simulink model "motion_with_control"  (R2020b)
settings: Solver=FixedStepDiscrete  StartTime=0.0  StopTime=inf  FixedStep=0.001  RelTol=1e-3  EnableMultiTasking=on
PreLoadFcn:
  | demos_common_configs();
undefined symbols (not defined in the file): DiscIntNeverNeededParam
libraries: franka_simulink_library_misc x5, franka_simulink_library x4
settings Model: SimulationMode=external  ExtModeTrigDuration=10000  Creator=vasi_ko  LastModifiedBy=kvasios
settings DataIOCC: LimitDataPoints=on  SaveFormat=Array  ReturnWorkspaceOutputs=off
settings OptimizationCC: DefaultParameterBehavior=Inlined  EnhancedBackFolding=on  PassReuseOutputArgsAs=Individual arguments  ZeroExternalMemoryAtStartup=off  ZeroInternalMemoryAtStartup=off  OptimizeBlockOrder=speed  DifferentSizesBufferReuse=on  OptimizationCustomize=off  EfficientTunableParamExpr=on
settings DebuggingCC: SolverPrmCheckMsg=warning  ParameterTunabilityLossMsg=error  SFUnexpectedBacktrackingDiag=warning  SFNoUnconditionalDefaultTransitionDiag=warning  SFExecutionAtInitializationDiag=none  ArithmeticOperatorsInVariantConditions=warning
settings HardwareCC: ProdBitPerLong=64  ProdHWDeviceType=Intel->x86-64 (Linux 64)
settings ModelReferenceCC: PropagateSignalLabelsOutOfModel=off
settings SFSimCC: SimUseLocalCustomCode=off  MATLABDynamicMemAlloc=off  CustomCodeUndefinedFunction=UseInterfaceOnly  SimTargetLang=C++
settings RTWCC: Description=Embedded Coder  SystemTargetFile=franka_emika_panda.tlc  GenCodeOnly=on  TemplateMakefile=ert_default_tmf  RTWVerbose=off  RTWUseLocalCustomCode=off  Toolchain=Franka Simulink | gmake (64-bit linux)  BuildConfiguration=Faster Runs  IncludeHyperlinkInReport=on  TargetLang=C++
settings CodeAppCC: ForceParamTrailComments=on  IgnoreCustomStorageClasses=off  OperatorAnnotations=on  SimulinkDataObjDesc=on  SFDataObjDesc=on  InsertBlockDesc=on
settings STFCustomTargetCC: TargetLangStandard=C99 (ISO)  MultiwordLength=256  GenerateSampleERTMain=on  ModelReferenceCompliant=off  ConcurrentExecutionCompliant=off  CombineOutputUpdateFcns=on  ERTCustomFileBanners=on  SupportNonInlinedSFcns=off  RemoveResetFunc=on  MATLABClassNameForMDSCustomization=Simulink.SoftwareTarget.ERTCustomization  GRTInterface=off  UseToolchainInfoCompliant=on  SystemTargetFile=franka_emika_panda.tlc
settings ERTTargetCC: TargetLangStandard=C99 (ISO)  GenerateSampleERTMain=on  ModelReferenceCompliant=off  ParMdlRefBuildCompliant=off  CompOptLevelCompliant=off  ConcurrentExecutionCompliant=off  SupportContinuousTime=on  ModelStepFunctionPrototypeControlCompliant=off  InlinedParameterPlacement=NonHierarchical  ERTCustomFileTemplate=franka_emika_panda_file_process.tlc
settings ConfigComp: CovMetricSettings=dw  CovSaveCumulativeToWorkspaceVar=on  CovSaveSingleToWorkspaceVar=on  CovExternalEMLEnable=off  CovSFcnEnable=off

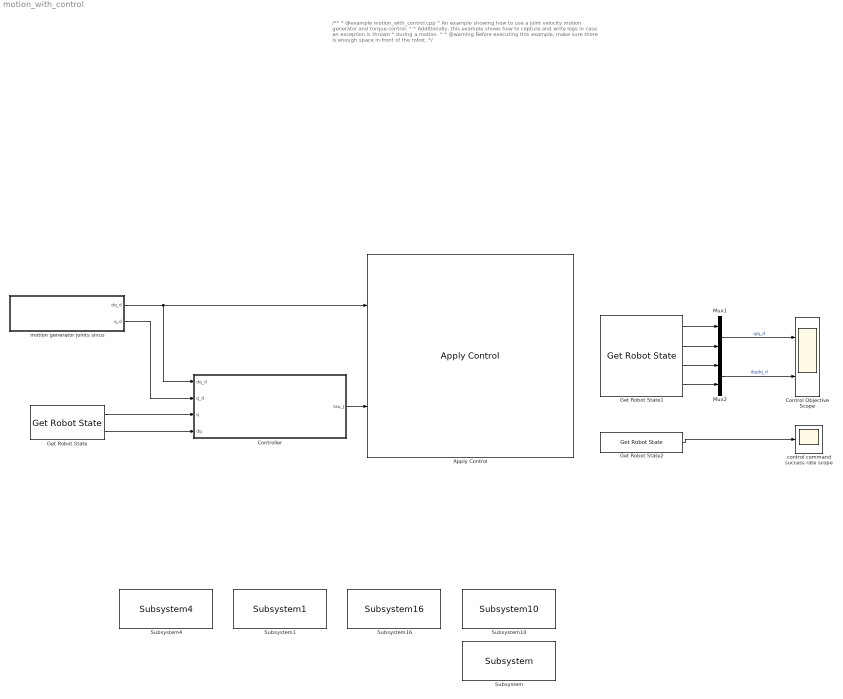
== system motion_with_control ==
  note: /**
      |  * @example motion_with_control.cpp
      |  * An example showing how to use a joint velocity motion generator and torque control.
      |  *
      |  * Additionally, this example shows how to capture and write logs in case an exception is thrown
      |  * during a motion.
      |  *
      |  * @warning Before executing this example, make sure there is enough space in front of the robot.
      |  */
  Apply Control : franka_simulink_library/Apply Control  robot_ip=robot_ip  gripper_attached=off  control_mode=Torque Control - Joint Velocities  controller_choice=Joint Impedance Controller  elbow_control=on  collision_thresholds=collision_behavior  joint_impedance=joint_impedance  cartesian_impedance=cartesian_impedance  load_inertia=load_inertia  EE_T_K=EE_T_K  init_joint_configuration_req=on  init_joint_configuration=q_init
      settings: SourceProductName=Franka Emika
  Control Objective Scope : Scope  NumInputPorts=2
  Controller : Subsystem
      mask Display:
      | % pos = get_param(gcb, 'Position');
      | 
      | disp('{\bf\fontsize{18}PD Controller}', 'texmode','on');
      | 
      | block_icon('Controller')
      | 
      | port_label('output',1,'tau_J_d');
      | 
      | port_label('input',2,'q_d');
      | port_label('input',1,'dq_d');
      | port_label('input',3,'q');
      | port_label('input',4,'dq');
  Get Robot State : franka_simulink_library/Get Robot State  robot_ip=robot_ip  signals_requested='q dq'
      settings: SourceProductName=Franka Emika
  Get Robot State1 : franka_simulink_library/Get Robot State  robot_ip=robot_ip  signals_requested='q q_d dq dq_d'
      settings: SourceProductName=Franka Emika
  Get Robot State2 : franka_simulink_library/Get Robot State  robot_ip=robot_ip  signals_requested='control_command_success_rate'
      settings: SourceProductName=Franka Emika
  Mux1 : Mux  Inputs=2
  Mux2 : Mux  Inputs=2
  Subsystem : franka_simulink_library_misc/Subsystem  SystemSampleTime=-1  VariantActivationTime=update diagram  Latency=0  AutoFrameSizeCalculation=off
  Subsystem1 : franka_simulink_library_misc/Subsystem1  SystemSampleTime=-1  VariantActivationTime=update diagram  Latency=0  AutoFrameSizeCalculation=off
  Subsystem10 : franka_simulink_library_misc/Subsystem10  SystemSampleTime=-1  VariantActivationTime=update diagram  Latency=0  AutoFrameSizeCalculation=off
  Subsystem16 : franka_simulink_library_misc/Subsystem16  SystemSampleTime=-1  VariantActivationTime=update diagram  Latency=0  AutoFrameSizeCalculation=off
  Subsystem4 : franka_simulink_library_misc/Subsystem4  SystemSampleTime=-1  VariantActivationTime=update diagram  Latency=0  AutoFrameSizeCalculation=off
  control command success rate scope : Scope
  motion generator joints sinus : Subsystem
      mask Display:
      | pos = get_param(gcb, 'Position');
      | width = pos(3) - pos(1);
      | x = [0:width];
      | y = sin(x/180*pi);
      | % Parameters 'm' and 'b' must be defined in 'Parameters & Dialog' pane.
      | plot(x,y );
      | 
      | port_label('output',1,'dq_d');
      | port_label('output',2,'q_d');
  wires:
  motion generator joints sinus/1(dq_d) -> Controller/1(dq_d), Apply Control/1
  motion generator joints sinus/2(q_d) -> Controller/2(q_d)
  Controller/1(tau_J) -> Apply Control/2
  Mux2/1 -> Control Objective Scope/2  "dq/dq_d"
  Get Robot State/2 -> Controller/4(dq)
  Mux1/1 -> Control Objective Scope/1  "q/q_d"
  Get Robot State/1 -> Controller/3(q)
  Get Robot State1/1 -> Mux1/1
  Get Robot State1/2 -> Mux1/2
  Get Robot State1/3 -> Mux2/1
  Get Robot State1/4 -> Mux2/2
  Get Robot State2/1 -> control command success rate scope/1

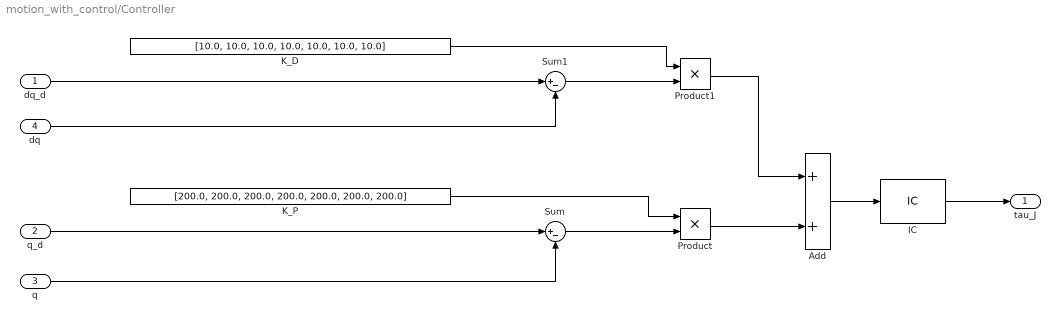
== system motion_with_control/Controller ==
  dq_d : Inport
  q_d : Inport  Port=2
  q : Inport  Port=3
  dq : Inport  Port=4
  Add : Sum
  IC : InitialCondition  Value=zeros(1,7)
  K_D : Constant  Value=[10.0, 10.0, 10.0, 10.0, 10.0, 10.0, 10.0]  VectorParams1D=off  SampleTime=-1
  K_P : Constant  Value=[200.0, 200.0, 200.0, 200.0, 200.0, 200.0, 200.0]  VectorParams1D=off  SampleTime=-1
  Product : Product
  Product1 : Product
  Sum : Sum  Inputs=|+-
  Sum1 : Sum  Inputs=|+-
  tau_J : Outport  VectorParamsAs1DForOutWhenUnconnected=off
  wires:
  IC/1 -> tau_J/1
  Add/1 -> IC/1
  Sum1/1 -> Product1/2
  dq/1 -> Sum1/2
  q_d/1 -> Sum/1
  dq_d/1 -> Sum1/1
  Product1/1 -> Add/1
  Product/1 -> Add/2
  K_D/1 -> Product1/1
  K_P/1 -> Product/1
  Sum/1 -> Product/2
  q/1 -> Sum/2

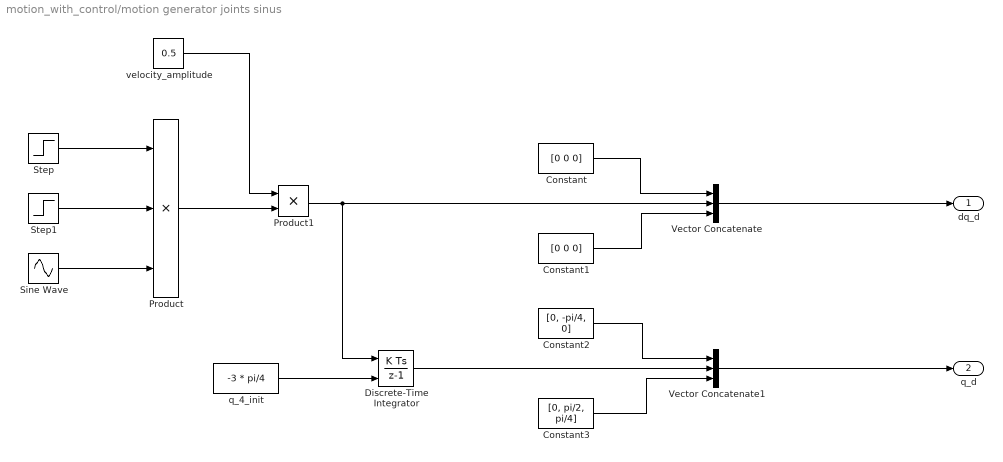
== system motion_with_control/motion generator joints sinus ==
  Constant : Constant  Value=[0 0 0]  VectorParams1D=off
  Constant1 : Constant  Value=[0 0 0]  VectorParams1D=off
  Constant2 : Constant  Value=[0, -pi/4, 0]  VectorParams1D=off
  Constant3 : Constant  Value=[0, pi/2, pi/4]  VectorParams1D=off
  Discrete-Time Integrator : DiscreteIntegrator  InitialConditionSource=external  SampleTime=0.001  ICPrevOutput=DiscIntNeverNeededParam  ICPrevScaledInput=DiscIntNeverNeededParam
  Product : Product  Inputs=3
  Product1 : Product
  Sine Wave : Sin  Frequency=pi  Phase=pi  SampleTime=0
  Step : Step  SampleTime=0
  Step1 : Step  Time=7  Before=1  After=0  SampleTime=0
  Vector Concatenate : Concatenate  NumInputs=3
  Vector Concatenate1 : Concatenate  NumInputs=3
  q_4_init : Constant  Value=-3 * pi/4  VectorParams1D=off
  velocity_amplitude : Constant  Value=0.5  VectorParams1D=off
  dq_d : Outport  VectorParamsAs1DForOutWhenUnconnected=off
  q_d : Outport  Port=2  VectorParamsAs1DForOutWhenUnconnected=off
  wires:
  Constant1/1 -> Vector Concatenate/3
  Constant/1 -> Vector Concatenate/1
  Product/1 -> Product1/2
  Sine Wave/1 -> Product/3
  Step/1 -> Product/1
  velocity_amplitude/1 -> Product1/1
  Product1/1 -> Discrete-Time Integrator/1, Vector Concatenate/2
  Vector Concatenate/1 -> dq_d/1
  Constant3/1 -> Vector Concatenate1/3
  Constant2/1 -> Vector Concatenate1/1
  Discrete-Time Integrator/1 -> Vector Concatenate1/2
  Vector Concatenate1/1 -> q_d/1
  q_4_init/1 -> Discrete-Time Integrator/2
  Step1/1 -> Product/2
